simulink model "propeller_combined_feedback_feedforward_start"  (R2021b)
settings: Solver=VariableStepAuto  StartTime=0.0  StopTime=Inf  RelTol=1e-3
settings Model: Creator=cirie  LastModifiedBy=cirie

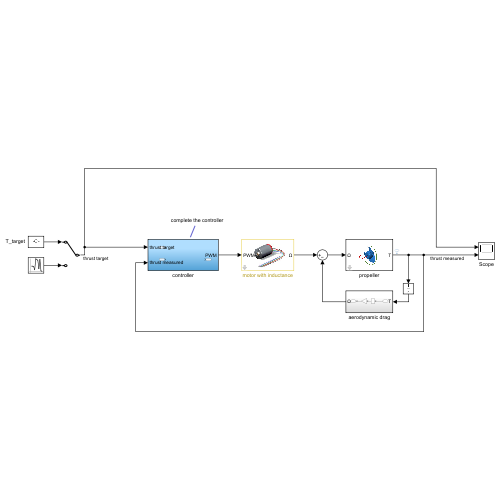
[thumbnail: Simulink's stored preview of the top-level diagram]
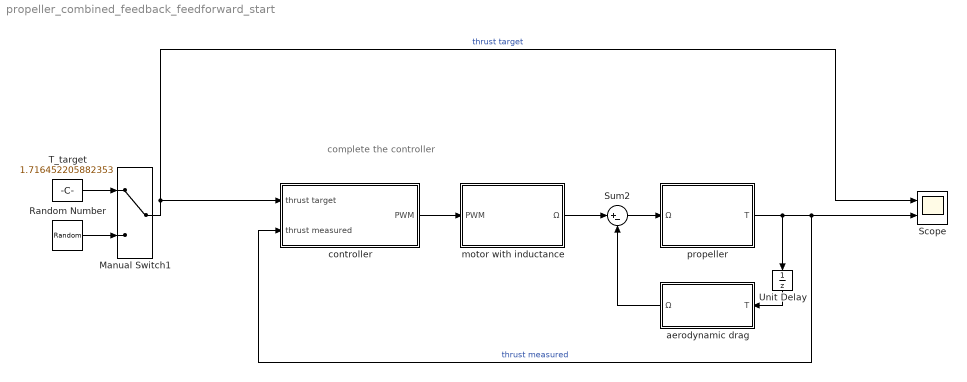
== system propeller_combined_feedback_feedforward_start ==
  note: complete the controller
  Manual Switch1 : ManualSwitch
  Random Number : RandomNumber  Mean=1  Variance=0.25  SampleTime=1
  Scope : Scope  NumInputPorts=2
  Sum2 : Sum  Inputs=|+-
  T_target : Constant  Value=1.716452205882353
  Unit Delay : UnitDelay  SampleTime=1e-3  HasFrameUpgradeWarning=on
  aerodynamic drag : Subsystem
  controller : Subsystem
  motor with inductance : Subsystem  mask(DC Motor){J=1e-4, km=0.1, R=1, L=1e-3, Vmax=7.2}
      mask prompts: J "Inertia, J [kgm^2]"; km "Motor constant, km [V*s/rad]"; R "Resistance, R [Ohm]"; L "Inductance, L [H]"; Vmax "Maximum Voltage, Vmax [V]"
      mask help:
      | Circuit Dynamics:   PWM*Vmax == I*R + km*Ω
      | Rotor Dynamics:     J*dΩ/dt == km*I
      mask Display: image('$imagefile'); % Use "Edit Image" on toolstrip to change.
  propeller : Subsystem  mask(Propeller Model){D=0.1, kt=0.01, rho=1000}
      mask prompts: D "Propeller Diameter [m]"; kt "Thrust Coefficient"; rho "Fluid density [kg/m^3]"
      mask help: Propeller Dynamics: T = kt*rho*omega^2*D^4
      mask Display: image('$imagefile'); % Use "Edit Image" on toolstrip to change.
  wires:
  propeller/1(T) -> Unit Delay/1, controller/2(thrust measured), Scope/2  "thrust measured"
  Manual Switch1/1 -> Scope/1, controller/1(thrust target)  "thrust target"
  motor with inductance/1(Ω) -> Sum2/1
  Random Number/1 -> Manual Switch1/2
  T_target/1 -> Manual Switch1/1
  aerodynamic drag/1(Ω) -> Sum2/2
  Unit Delay/1 -> aerodynamic drag/1(T)
  Sum2/1 -> propeller/1(Ω)
  controller/1(PWM) -> motor with inductance/1(PWM)

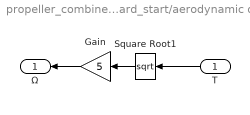
== system propeller_combined_feedback_feedforward_start/aerodynamic drag ==
  T : Inport
  Gain : Gain  Gain=5
  Square Root1 : Sqrt  SaturateOnIntegerOverflow=on
  Ω : Outport
  wires:
  Square Root1/1 -> Gain/1
  T/1 -> Square Root1/1
  Gain/1 -> Ω/1

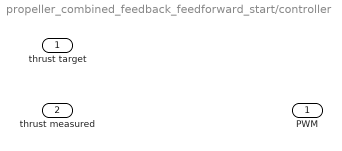
== system propeller_combined_feedback_feedforward_start/controller ==
  thrust target : Inport
  thrust measured : Inport  Port=2
  PWM : Outport

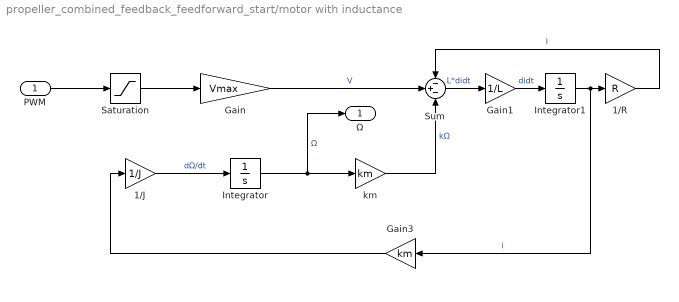
== system propeller_combined_feedback_feedforward_start/motor with inductance ==
  PWM : Inport
  1/J : Gain  Gain=1/J
  1/R : Gain  Gain=R
  Gain : Gain  Gain=Vmax
  Gain1 : Gain  Gain=1/L
  Gain3 : Gain  Gain=km
  Integrator : Integrator
  Integrator1 : Integrator
  Saturation : Saturate  UpperLimit=1  LowerLimit=-1
  Sum : Sum  Inputs=-+-
  km : Gain  Gain=km
  Ω : Outport
  wires:
  1/J/1 -> Integrator/1  "dΩ/dt"
  Integrator1/1 -> Gain3/1, 1/R/1  "i"
  Integrator/1 -> Ω/1, km/1  "Ω"
  Gain3/1 -> 1/J/1
  km/1 -> Sum/3  "kΩ"
  1/R/1 -> Sum/1  "I"
  PWM/1 -> Saturation/1
  Gain/1 -> Sum/2  "V"
  Saturation/1 -> Gain/1
  Sum/1 -> Gain1/1  "L*didt"
  Gain1/1 -> Integrator1/1  "didt"

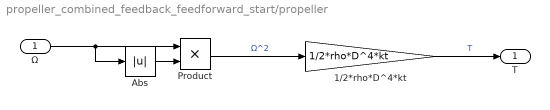
== system propeller_combined_feedback_feedforward_start/propeller ==
  Ω : Inport
  1/2*rho*D^4*kt : Gain  Gain=1/2*rho*D^4*kt
  Abs : Abs
  Product : Product
  T : Outport
  wires:
  1/2*rho*D^4*kt/1 -> T/1  "T"
  Product/1 -> 1/2*rho*D^4*kt/1  "Ω^2"
  Ω/1 -> Abs/1, Product/1
  Abs/1 -> Product/2
